simulink model "MPC_Quad_4SV_backup_before_refine"  (R2022b)
settings: Solver=FixedStepAuto  StartTime=0.0  StopTime=30  FixedStep=Ts  RelTol=1e-3
undefined symbols (not defined in the file): A, B, C, Cm, Ct, D, estim_hover_nrpm, g, initState, Ir, Ixx, Iyy, Izz, Length, mass
libraries: uavutilslib x2, sharedtransform x1, mpclib x1
settings Model: PacingRate=0.350000  Creator=Bw Jiang  LastModifiedBy=Bw Jiang
settings DebuggingCC: AlgebraicLoopMsg=none  ParameterOverflowMsg=none  ParameterUnderflowMsg=error

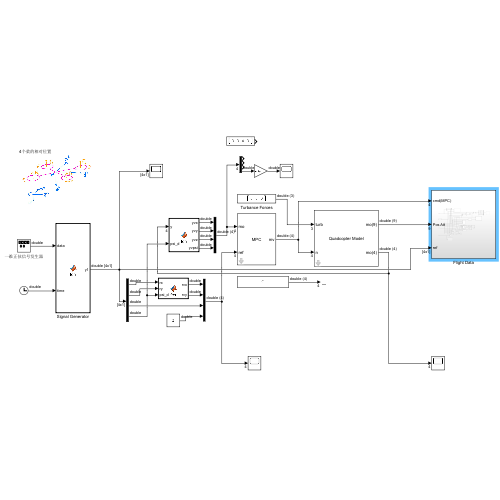
[thumbnail: Simulink's stored preview of the top-level diagram]
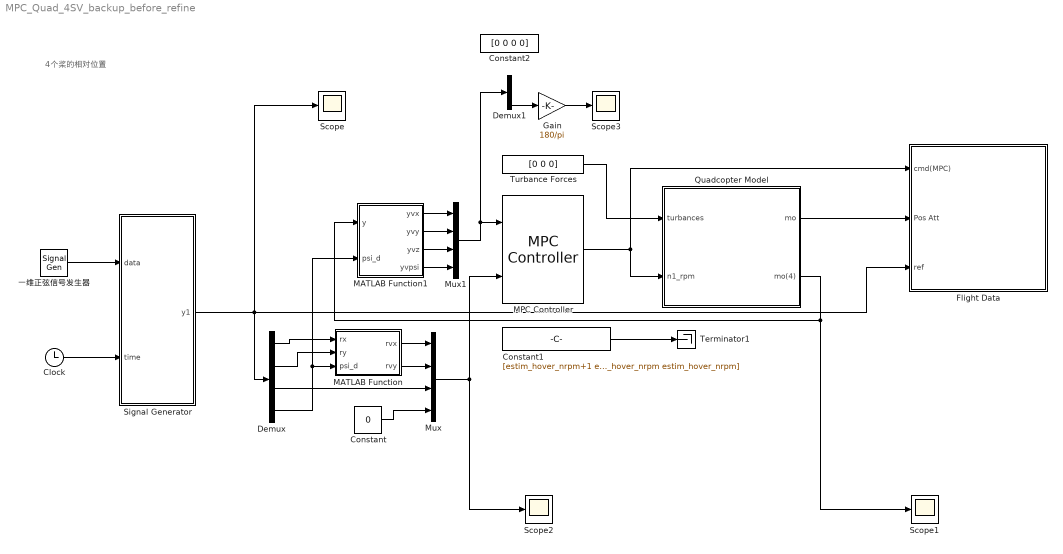
== system MPC_Quad_4SV_backup_before_refine ==
  note: 4个桨的相对位置
  Clock : Clock
  Constant : Constant  Value=0
  Constant1 : Constant  Value=[estim_hover_nrpm+1 estim_hover_nrpm estim_hover_nrpm estim_hover_nrpm]
  Constant2 : Constant  Value=[0 0 0 0]
  Demux : Demux
  Demux1 : Demux
  Flight Data : Subsystem
  Gain : Gain  Gain=180/pi
  MATLAB Function : MATLAB Function  TreatAsAtomicUnit=on
  MATLAB Function1 : MATLAB Function  TreatAsAtomicUnit=on
  MPC Controller : mpclib/MPC Controller  SCDEnableBlockLinearizationSpecification=on  mpcobj=mpc4sv  is_multiple=0  enable_value=0  return_u0=off  updateMPCinCallerWorkspace=on  md_inport=off  mv_inport=off  uref_inport=off  return_cost=off  return_mvseq=off  return_qpstatus=off  return_xseq=off  return_state=off  return_ovseq=off  state_inport=off  umin_inport=off  umax_inport=off  ymin_inport=off  ymax_inport=off  cc_inport=off  ywt_inport=off  uwt_inport=off  duwt_inport=off  rhoeps_inport=off  pm_inport=off  MaximumP=10  HorizonChoice=FixedHorizon  n_ts=0.05  n_p=30  n_mv=4  n_md=0  n_ud=0  n_mo=4  n_uo=0  BlockDataType=double  SampleTimeInherited=off  switch_inport=off
  Mux : Mux
  Mux1 : Mux
  Quadcopter Model : Subsystem  mask{g=g, mass=mass, I_xx=Ixx, I_yy=Iyy, I_zz=Izz, I_r=Ir, L=Length, C_M=Cm, C_T=Ct}
      mask prompts: g "Gravity"; I_xx "Inertia_xx"; I_yy "Inertia_yy"; I_zz "Inertia_zz"; I_r "Inertia_per_rotor"; L "Length"
      mask DialogControl ParameterGroupVar Prompt: 参数
      mask Display:
      | disp('Quadcopter Model');
      | port_label('input', 1, 'turb')
      | port_label('input', 2, 'n')
      | % port_label('input', 3, 'n3')
      | % port_label('input', 4, 'n4')
      | port_label('output', 1, 'mo(9)')
      | port_label('output', 2, 'mo(4)')
      | % port_label('output', 3, 'y')
      | % port_label('output', 4, 'vy')
      | % port_label('output', 5, 'z')
      | % port_label('output', 6, 'vz')
      | % port_label('output', 7, 'phi')
      | % port_label('output', 8, 'd_phi')
      | % port_label('output', 9, 'theta')
      | % port_label('output', 10, 'd_theta')
      | % port_label('output', 11, 'psi')
      | % port_label('output', 12, 'd_psi')
  Scope{,1..3} (4 alike) : Scope
  Signal Generator : MATLAB Function  TreatAsAtomicUnit=on
  Terminator1 : Terminator
  Turbance Forces : Constant  Value=[0 0 0]
  一维正弦信号发生器 : SignalGenerator  Frequency=0.01
  wires:
  Clock/1 -> Signal Generator/2(time)
  MPC Controller/1 -> Flight Data/1(cmd(MPC)), Quadcopter Model/2(n1_rpm)
  Constant1/1 -> Terminator1/1
  Quadcopter Model/1(mo) -> Flight Data/2(Pos Att)
  Quadcopter Model/2(mo(4)) -> MATLAB Function1/1(y), Scope1/1
  一维正弦信号发生器/1 -> Signal Generator/1(data)
  Turbance Forces/1 -> Quadcopter Model/1(turbances)
  Signal Generator/1(y1) -> Flight Data/3(ref), Demux/1, Scope/1
  Demux/3 -> Mux/3
  Constant/1 -> Mux/4
  Demux/1 -> MATLAB Function/1(rx)
  Demux/2 -> MATLAB Function/2(ry)
  Demux/4 -> MATLAB Function1/2(psi_d), MATLAB Function/3(psi_d)
  MATLAB Function/1(rvx) -> Mux/1
  MATLAB Function/2(rvy) -> Mux/2
  Mux/1 -> MPC Controller/2, Scope2/1
  MATLAB Function1/1(yvx) -> Mux1/1
  MATLAB Function1/2(yvy) -> Mux1/2
  MATLAB Function1/3(yvz) -> Mux1/3
  MATLAB Function1/4(yvpsi) -> Mux1/4
  Mux1/1 -> Demux1/1, MPC Controller/1
  Demux1/4 -> Gain/1
  Gain/1 -> Scope3/1

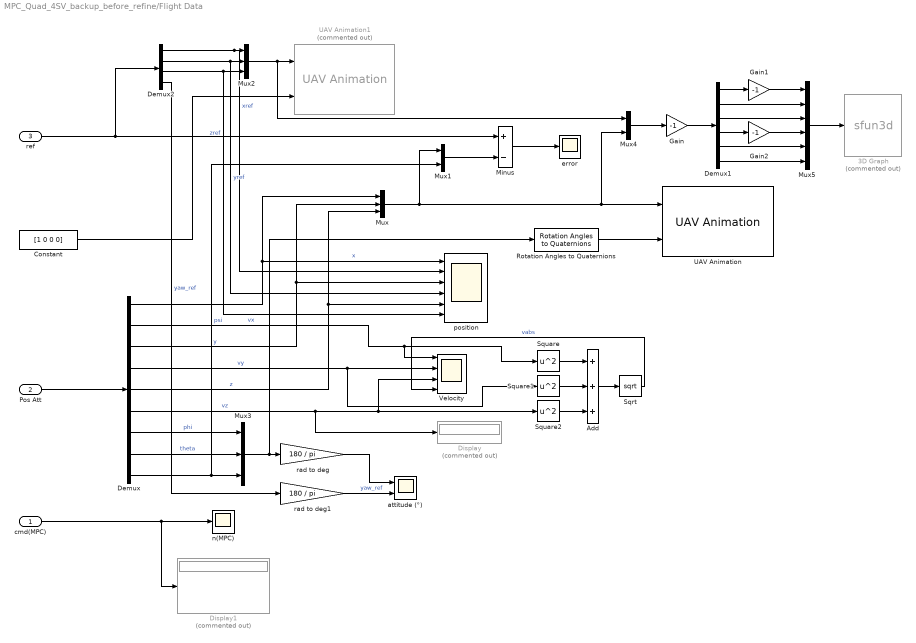
== system MPC_Quad_4SV_backup_before_refine/Flight Data ==
  cmd(MPC) : Inport
  Pos Att : Inport  Port=2
  ref : Inport  Port=3
  3D Graph : S-Function  Commented=on  LoadFcn=if exist('sfun3d','file'), sfun3d([],[],[],'LoadBlock'); end  FunctionName=sfun3d  Parameters=ax,T,np,cp,gd,ls,mk,mx,hd,tb  SFunctionDeploymentMode=off  EnableBusSupport=off  mask(3D Graph){np=2, ax=[-20 10 -10 10 -20 5], mx=50000, T=0.1, cp=[20 40 30], gd=on, hd=on, tb=on, ls=-, mk=none}
      mask prompts: np "Number of moving points (lines)"; ax "Range: [xmin xmax  ymin ymax zmin zmax]"; mx "Max number of points in each line"; T "Sampling Time"; cp "Camera position (use [0 0 1] for 2D XY view)"; gd "Grid (on|off)"; hd "HeadMarkers (on|off)"; tb "Toolbar (on|off)"; ls "LineStyle"; mk "LineMarker"
      mask help:
      | This block plots the position of several points in the XYZ space. The input contains the coordinates of all the points (x1,y1,z1,x2,y2,z2,...).
      | The number of moving points (lines), the XYZ ranges, sampling time, camera position, and grid (among other things) can be set as mask parameters.
      settings: CopyFcn=if exist('sfun3d','file'), sfun3d([],[],[],'CopyBlock'); end  DeleteFcn=if exist('sfun3d','file'), sfun3d([],[],[],'DeleteBlock'); end  NameChangeFcn=if exist('sfun3d','file'), sfun3d([],[],[],'NameChange'); end
      mask Help:
      | This block plots the position of several points in the XYZ space. The input contains the coordinates of all the points (x1,y1,z1,x2,y2,z2,...).
      | The number of moving points (lines), the XYZ ranges, sampling time, camera position, and grid (among other things) can be set as mask parameters.
      mask TypeOptions ls: - | -- | : | -. | none
      mask TypeOptions mk: none | . | + | o | * | x | square | diamond | v | ^ | > | < | pentagram | hexagram
      mask Display: plot([.05 .95 .95 .05 .05],[.45 .45 .95 .95 .45], 0.5+cos(0:0.1:2*pi)*0.3,0.7+sin(0:0.1:2*pi)*0.2)
  Add : Sum  Inputs=+++
  Constant : Constant  Value=[1 0 0 0]
  Demux : Demux  Outputs=9
  Demux1 : Demux  Outputs=6
  Demux2 : Demux
  Display : Display  Commented=on
  Display1 : Display  Commented=on
  Gain : Gain  Gain=-1
  Gain1 : Gain  Gain=-1
  Gain2 : Gain  Gain=-1
  Minus : Sum  Inputs=+-
  Mux : Mux  Inputs=3
  Mux1 : Mux  Inputs=2
  Mux2 : Mux  Inputs=3
  Mux3 : Mux  Inputs=3
  Mux4 : Mux  Inputs=2
  Mux5 : Mux  Inputs=6
  Rotation Angles to Quaternions : sharedtransform/Rotation Angles to Quaternions  rotationOrder=XYZ  aMode=aMode
  Sqrt : Sqrt
  Square : Math  Operator=square
  Square1 : Math  Operator=square
  Square2 : Math  Operator=square
  UAV Animation : uavutilslib/UAV Animation  UAVType=Multirotor  UAVSize=1  InertialZDirection=Down  SampleTime=-1
  UAV Animation1 : uavutilslib/UAV Animation  Commented=on  UAVType=Multirotor  UAVSize=1  InertialZDirection=Down  SampleTime=-1
  Velocity : Scope  NumInputPorts=4
  attitude (°) : Scope  NumInputPorts=2
  error : Scope
  n(MPC) : Scope
  position : Scope  NumInputPorts=6
  rad to deg : Gain  Gain=180 / pi
  rad to deg1 : Gain  Gain=180 / pi
  wires:
  Demux/8 -> Mux3/2  "theta"
  Demux/4 -> Square1/1, Velocity/2  "vy"
  Demux/2 -> Velocity/1, Square/1  "vx"
  Demux/7 -> Mux3/1  "phi"
  Demux/6 -> Velocity/3, Square2/1, Display/1  "vz"
  Demux/5 -> Mux/3, position/5  "z"
  Demux/1 -> Mux/1, position/1  "x"
  Demux/3 -> position/3, Mux/2  "y"
  rad to deg/1 -> attitude (°)/1
  Mux3/1 -> Rotation Angles to Quaternions/1, rad to deg/1
  cmd(MPC)/1 -> n(MPC)/1, Display1/1
  Pos Att/1 -> Demux/1
  Demux/9 -> Mux1/2, Mux3/3  "psi"
  Mux/1 -> Mux4/2, UAV Animation/1, Mux1/1
  Constant/1 -> UAV Animation1/2
  Mux1/1 -> Minus/2
  Minus/1 -> error/1
  ref/1 -> Demux2/1, Minus/1
  Demux2/1 -> position/2, Mux2/1  "xref"
  Demux2/2 -> position/4, Mux2/2  "yref"
  Demux2/3 -> position/6, Mux2/3  "zref"
  Mux2/1 -> Mux4/1, UAV Animation1/1
  Square/1 -> Add/1
  Square1/1 -> Add/2
  Square2/1 -> Add/3
  Add/1 -> Sqrt/1
  Sqrt/1 -> Velocity/4  "vabs"
  Mux4/1 -> Gain/1
  Gain/1 -> Demux1/1
  Demux1/1 -> Gain1/1
  Demux1/4 -> Gain2/1
  Gain1/1 -> Mux5/1
  Demux1/2 -> Mux5/2
  Demux1/3 -> Mux5/3
  Gain2/1 -> Mux5/4
  Demux1/5 -> Mux5/5
  Demux1/6 -> Mux5/6
  Mux5/1 -> 3D Graph/1
  Demux2/4 -> rad to deg1/1  "yaw_ref"
  rad to deg1/1 -> attitude (°)/2  "yaw_ref"
  Rotation Angles to Quaternions/1 -> UAV Animation/2

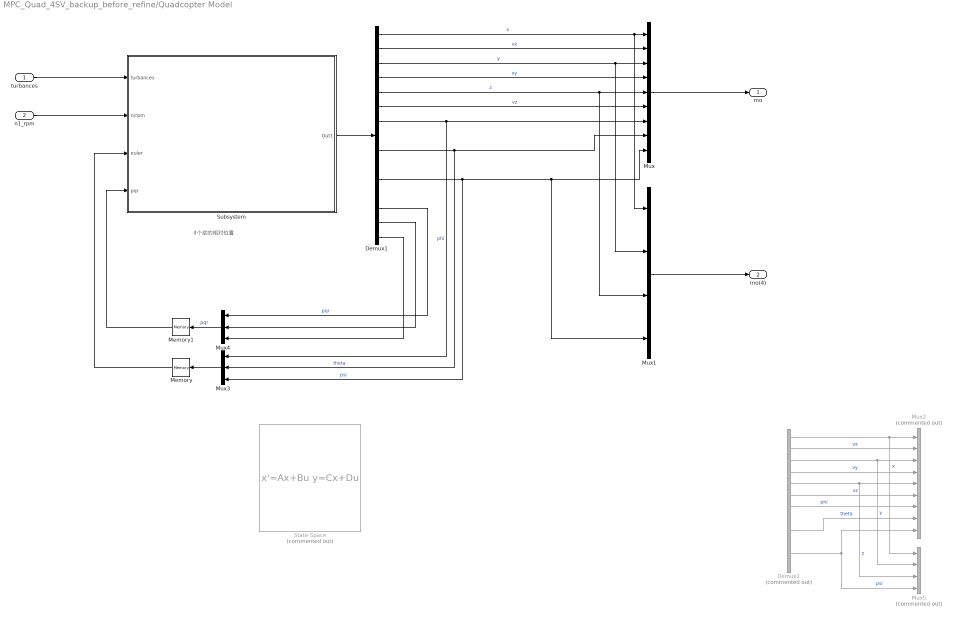
== system MPC_Quad_4SV_backup_before_refine/Quadcopter Model ==
  note: 4个桨的相对位置
  turbances : Inport
  n1_rpm : Inport  Port=2
  Demux1 : Demux  Outputs=15
  Demux2 : Demux  Commented=on  Outputs=12
  Memory : Memory  InheritSampleTime=on
  Memory1 : Memory  InheritSampleTime=on
  Mux : Mux  Inputs=9
  Mux1 : Mux
  Mux2 : Mux  Commented=on  Inputs=9
  Mux3 : Mux  Inputs=3
  Mux4 : Mux  Inputs=3
  Mux5 : Mux  Commented=on
  State-Space : StateSpace  Commented=on  A=A  B=B  C=C  D=D  InitialCondition=0
  Subsystem : Subsystem
  mo : Outport
  mo(4) : Outport  Port=2
  wires:
  n1_rpm/1 -> Subsystem/2(n/rpm)
  Memory1/1 -> Subsystem/4(pqr)
  Demux1/15 -> Mux4/3
  Demux1/13 -> Mux4/1  "pqr"
  Mux4/1 -> Memory1/1  "pqr"
  Demux1/9 -> Mux/8, Mux3/2  "theta"
  Demux1/1 -> Mux1/1, Mux/1  "x"
  Demux1/2 -> Mux/2  "vx"
  Demux1/11 -> Mux1/4, Mux/9, Mux3/3  "psi"
  Demux1/4 -> Mux/4  "vy"
  Demux1/3 -> Mux1/2, Mux/3  "y"
  Demux1/5 -> Mux1/3, Mux/5  "z"
  Subsystem/1(Out1) -> Demux1/1
  Memory/1 -> Subsystem/3(euler)
  Demux1/6 -> Mux/6  "vz"
  Demux1/7 -> Mux/7, Mux3/1  "phi"
  Mux3/1 -> Memory/1
  Demux1/14 -> Mux4/2
  turbances/1 -> Subsystem/1(turbances)
  Demux2/1 -> Mux2/1, Mux5/1  "x"
  Demux2/2 -> Mux2/2  "vx"
  Demux2/3 -> Mux5/2, Mux2/3  "y"
  Demux2/4 -> Mux2/4  "vy"
  Demux2/5 -> Mux5/3, Mux2/5  "z"
  Demux2/6 -> Mux2/6  "vz"
  Demux2/7 -> Mux2/7  "phi"
  Demux2/9 -> Mux2/8  "theta"
  Demux2/11 -> Mux5/4, Mux2/9  "psi"
  Mux/1 -> mo/1
  Mux1/1 -> mo(4)/1

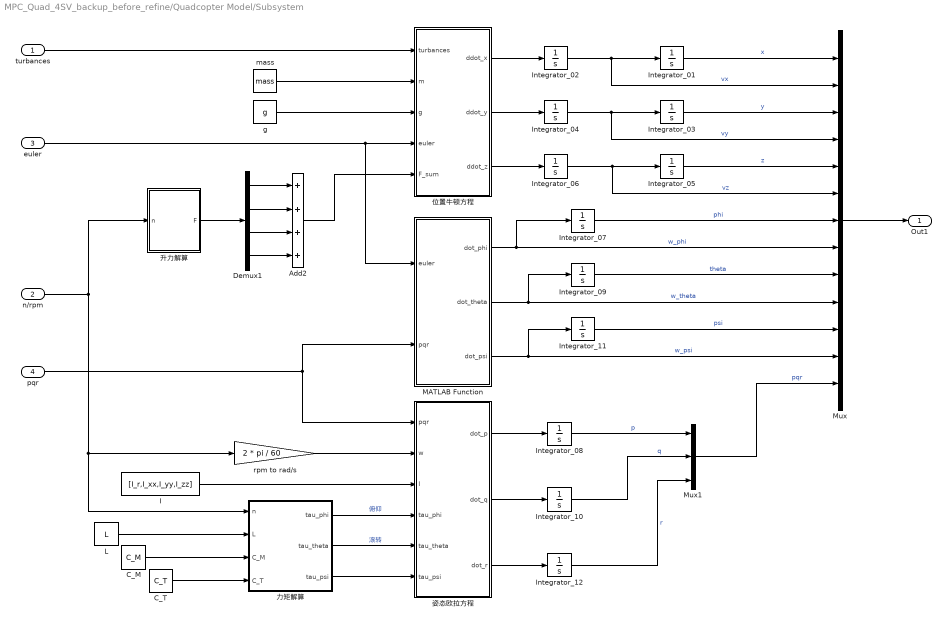
== system MPC_Quad_4SV_backup_before_refine/Quadcopter Model/Subsystem ==
  turbances : Inport
  n/rpm : Inport  Port=2  PortDimensions=4
  euler : Inport  Port=3  PortDimensions=3
  pqr : Inport  Port=4  PortDimensions=3
  Add2 : Sum  Inputs=++++
  C_M : Constant  Value=C_M
  C_T : Constant  Value=C_T
  Demux1 : Demux
  I : Constant  Value=[I_r,I_xx,I_yy,I_zz]
  Integrator_01 : Integrator  InitialCondition=initState.x
  Integrator_02 : Integrator  InitialCondition=initState.vx
  Integrator_03 : Integrator  InitialCondition=initState.y
  Integrator_04 : Integrator  InitialCondition=initState.vy
  Integrator_05 : Integrator  InitialCondition=initState.z
  Integrator_06 : Integrator  InitialCondition=initState.vz
  Integrator_07 : Integrator  InitialCondition=initState.phi
  Integrator_08 : Integrator  InitialCondition=initState.p
  Integrator_09 : Integrator  InitialCondition=initState.theta
  Integrator_10 : Integrator  InitialCondition=initState.q
  Integrator_11 : Integrator  InitialCondition=initState.psi
  Integrator_12 : Integrator  InitialCondition=initState.r
  L : Constant  Value=L
  MATLAB Function : MATLAB Function  TreatAsAtomicUnit=on
  Mux : Mux  Inputs=13
  Mux1 : Mux  Inputs=3
  g : Constant  Value=g
  mass : Constant  Value=mass
  rpm to rad/s : Gain  Gain=2 * pi / 60
  位置牛顿方程 : MATLAB Function  TreatAsAtomicUnit=on
  力矩解算 : MATLAB Function  TreatAsAtomicUnit=on
  升力解算 : MATLAB Function  TreatAsAtomicUnit=on
  姿态欧拉方程 : MATLAB Function  TreatAsAtomicUnit=on
  Out1 : Outport
  wires:
  姿态欧拉方程/1(dot_p) -> Integrator_08/1
  Demux1/4 -> Add2/4
  pqr/1 -> MATLAB Function/2(pqr), 姿态欧拉方程/1(pqr)
  位置牛顿方程/2(ddot_y) -> Integrator_04/1
  姿态欧拉方程/2(dot_q) -> Integrator_10/1
  I/1 -> 姿态欧拉方程/3(I)
  位置牛顿方程/3(ddot_z) -> Integrator_06/1
  Mux/1 -> Out1/1
  g/1 -> 位置牛顿方程/3(g)
  位置牛顿方程/1(ddot_x) -> Integrator_02/1
  Integrator_10/1 -> Mux1/2  "q"
  Demux1/1 -> Add2/1
  力矩解算/1(tau_phi) -> 姿态欧拉方程/4(tau_phi)  "俯仰"
  Integrator_08/1 -> Mux1/1  "p"
  euler/1 -> MATLAB Function/1(euler), 位置牛顿方程/4(euler)
  Integrator_03/1 -> Mux/3  "y"
  Integrator_09/1 -> Mux/9  "theta"
  力矩解算/3(tau_psi) -> 姿态欧拉方程/6(tau_psi)
  Demux1/2 -> Add2/2
  Add2/1 -> 位置牛顿方程/5(F_sum)
  Integrator_12/1 -> Mux1/3  "r"
  mass/1 -> 位置牛顿方程/2(m)
  力矩解算/2(tau_theta) -> 姿态欧拉方程/5(tau_theta)  "滚转"
  Demux1/3 -> Add2/3
  Integrator_05/1 -> Mux/5  "z"
  Integrator_01/1 -> Mux/1  "x"
  Integrator_02/1 -> Integrator_01/1, Mux/2  "vx"
  Integrator_07/1 -> Mux/7  "phi"
  Integrator_04/1 -> Mux/4, Integrator_03/1  "vy"
  Integrator_06/1 -> Mux/6, Integrator_05/1  "vz"
  Integrator_11/1 -> Mux/11  "psi"
  姿态欧拉方程/3(dot_r) -> Integrator_12/1
  MATLAB Function/3(dot_psi) -> Integrator_11/1, Mux/12  "w_psi"
  MATLAB Function/2(dot_theta) -> Integrator_09/1, Mux/10  "w_theta"
  MATLAB Function/1(dot_phi) -> Integrator_07/1, Mux/8  "w_phi"
  Mux1/1 -> Mux/13  "pqr"
  升力解算/1(F) -> Demux1/1
  L/1 -> 力矩解算/2(L)
  n/rpm/1 -> 升力解算/1(n), rpm to rad/s/1, 力矩解算/1(n)
  rpm to rad/s/1 -> 姿态欧拉方程/2(w)
  C_M/1 -> 力矩解算/3(C_M)
  C_T/1 -> 力矩解算/4(C_T)
  turbances/1 -> 位置牛顿方程/1(turbances)

== matlab function MPC_Quad_4SV_backup_before_refine/Quadcopter Model/Subsystem/MATLAB Function ==
  data: euler input; pqr input; dot_phi output; dot_theta output; dot_psi output
function [dot_phi, dot_theta, dot_psi] = fcn(euler, pqr)

% 角加速度的坐标转换，从机体系b到惯性系e

p = pqr(1);
q = pqr(2);
r = pqr(3);

phi =euler(1);
theta = euler(2);
psi = euler(3);

mat = [
    1, tan(theta) * sin(phi), tan(theta) * cos(phi);
    0, cos(phi), -sin(phi);
    0, sin(phi) / cos(theta), cos(phi) / cos(theta)
    ];
body = [p; q; r];
earth = mat * body;

dot_phi = earth(1);
dot_theta = earth(2);
dot_psi = earth(3);

== matlab function MPC_Quad_4SV_backup_before_refine/Quadcopter Model/Subsystem/位置牛顿方程 ==
  data: turbances input; m input; g input; euler input; ddot_x output; F_sum input; ddot_y output; ddot_z output
function [ddot_x, ddot_y, ddot_z] = fcn(turbances, m, g, euler, F_sum)

% F_sum恒正

phi =euler(1);
theta = euler(2);
psi = euler(3);

ddot_x = -((cos(phi) * sin(theta) * cos(psi) + sin(phi) * sin(psi)) * F_sum + turbances(1)) / m;
ddot_y = -((cos(phi) * sin(theta) * sin(psi) - sin(phi) * cos(psi)) * F_sum + turbances(2)) / m;
ddot_z = -(cos(phi) * cos(theta) * F_sum + turbances(3)) / m + g;

end

== matlab function MPC_Quad_4SV_backup_before_refine/Quadcopter Model/Subsystem/姿态欧拉方程 ==
  data: pqr input; dot_p output; w input; I input; dot_q output; dot_r output; tau_phi input; tau_theta input; tau_psi input
function [dot_p, dot_q, dot_r] = fcn(pqr, w, I, tau_phi, tau_theta, tau_psi)

w1 = w(1);
w2 = w(2);
w3 = w(3);
w4 = w(4);

p = pqr(1);
q = pqr(2);
r = pqr(3);

I_r = I(1);
I_xx = I(2);
I_yy = I(3);
I_zz = I(4);

w_tau = w1 - w2 + w3 - w4;

dot_p = (I_yy - I_zz) / I_xx * q * r - I_r * q / I_xx * w_tau + tau_phi / I_xx;
dot_q = (I_zz - I_xx) / I_yy * p * r + I_r * p / I_yy * w_tau + tau_theta / I_yy;
dot_r = (I_xx - I_yy) / I_zz * q * p + tau_psi / I_zz;

end

== matlab function MPC_Quad_4SV_backup_before_refine/Quadcopter Model/Subsystem/升力解算 ==
  data: n input; F output
function F = fcn(n)
%% Input Vars
% n - rpm

%% Output Vars
% F - N

%% Mid Vars
% omega - rad/s

%% Code

% F = n .* n * 2.414e-7 * 2;

omega = n / 60 * 2 * pi;
F = omega .* omega * 1.11e-5;

end

== matlab function MPC_Quad_4SV_backup_before_refine/Signal Generator ==
  data: data input; time input; y1 output
function y1  = fcn(data, time)

starttime = 2;

%% 悬停

% y1 = [0
%         0
%         0
%         0];

%% 螺旋线轨迹

% radspeed = 45; % 相当于相对圆心角的角速度 °/s
% vz = 0;
% r = 2 + time * 0.0;
% if time < starttime
%     y1 = [0
%           0
%           0
%           0];
% else
%     if r > 15
%         r = 15;
%     end
%     y1 = [r - r * cos(radspeed * (time - starttime) * pi / 180)
%           r * sin(radspeed * (time - starttime) * pi / 180)
%           -vz * time
%           0];
% end

%% 类8字轨迹

% radspeed = 10; % 相当于相对圆心角的角速度 °/s
% vz = 0.2;
% r1 = 4;
% r2 = 8;
% if time < starttime
%     y1 = [0; 0; 0; 0];
% else
%     if time < starttime + 180 / radspeed
%         y1 = [r1 - r1 * cos(radspeed * (time - starttime) * pi / 180)
%               r1 * sin(radspeed * (time - starttime) * pi / 180)
%               vz * (time - starttime)
%               0];
%     else
%         if time < starttime + 360 / radspeed
%             y1 = [-r2 * cos(radspeed * (time - starttime) * pi / 180)
%                   r2 * sin(radspeed * (time - starttime) * pi / 180)
%                   vz * (time - starttime)
%                   0];
%         else
%             if time < starttime + 540 / radspeed
%                 y1 = [-(r1 + r2) + r1 * cos(- radspeed * (time - starttime - 360 / radspeed) * pi / 180)
%                       r1 * sin(radspeed * (time - starttime) * pi / 180)
%                       vz * 360 / radspeed - vz * (time - starttime - 360 / radspeed)
%                       0];
%             else
%                 if time < starttime + 720 / radspeed
%                     y1 = [-r2 + r2 * cos(2 * pi - radspeed * (time - starttime - 360 / radspeed) * pi / 180)
%                           r2 * sin(radspeed * (time - starttime - 360 / radspeed) * pi / 180)
%                           vz * 360 / radspeed - vz * (time - starttime - 360 / radspeed)
%                           0];
%                 else
%                     y1 = [0; 0; 0; 0];
%                 end
%             end
%         end
%     end
% end

%% 阶跃轨迹

% x = 0;
% y = 0;
% z = 0;
% yaw = 0;
% 
% if time < 10
%     x = 0;
%     y = 0;
%     z = 0;
%     yaw = 0;
% elseif time > 10
%     x = 1;
%     y = 1.2;
%     z = -0.8;
%     yaw = 0;
% end
% 
% y1 = [x
%     y
%     z
%     yaw];

%% 偏航控制测试

yawspeed = 10; % °/s
yawspeed = yawspeed * pi / 180; % rad/s

t1 = starttime + 3;
t2 = t1 + 20;
t3 = t2 + 4;
t4 = t3 + 7;
t5 = t4 + 7;
if time < starttime
    y1 = [0
          0
          0
          0];
else
    if time < t1
    y1 = [0
          0
          0
          yawspeed * (time - starttime)];
    else
        if time < t2
            y1 = [0
                  0
                  0
                  yawspeed * (t1 - starttime)];
        else
            if time < t3
                y1 = [0
                      0
                      0
                      yawspeed * (time - t2 + t1 - starttime)];
            else
                if time < t4
                    y1 = [0
                          0
                          0
                          yawspeed * (t3 - t2 + t1 - starttime)];

                else
                    if time < t5
                        y1 = [0
                              0
                              0
                              yawspeed * (t3 - t2 + t1 - starttime) / (t4 - t5) * (time - t5)];
                    else
                        y1 = [0
                              0
                              0
                              0];
                    end
                end
            end
        end
    end
end

end

== matlab function MPC_Quad_4SV_backup_before_refine/Quadcopter Model/Subsystem/力矩解算 ==
  data: n input; L input; tau_phi output; tau_theta output; tau_psi output; C_M input; C_T input
function [tau_phi, tau_theta, tau_psi]= fcn(n, L, C_M, C_T)
%% Input Vars
% n - rpm
% L - m
% C_M - N*m*s^2/rad^2
% C_T - N*s^2/rad^2

%% Output Vars
% tau - N*m

%% Mid Vars
% w - rad/s

%% Code

% C_T = 1.1e-5;
% C_M = 1.0144e-7;

% F1 = F(1);
% F2 = F(2);
% F3 = F(3);
% F4 = F(4);

w1 = n(1) / 60 * 2 * pi;
w2 = n(2) / 60 * 2 * pi;
w3 = n(3) / 60 * 2 * pi;
w4 = n(4) / 60 * 2 * pi;

% I_r = I(1);

% w_tau = w1 + w3 - w2 - w4;

% 横滚
tau_phi = sqrt(2) / 2 * C_T * L * (w1^2 - w2^2 - w3^2 + w4^2); % tau_phi = (F1+F2-F3-F4) * L;
% 俯仰
tau_theta = sqrt(2) / 2 * C_T * L * (w1^2 + w2^2 - w3^2 - w4^2); % tau_theta = (F1-F2-F3+F4) * L;
% 偏航
tau_psi = C_M * (w1^2 - w2^2 + w3^2 - w4^2); % tau_psi = w_tau * I_r;

end

== matlab function MPC_Quad_4SV_backup_before_refine/MATLAB Function ==
  data: rx input; rvx output; ry input; psi_d input; rvy output
function [rvx, rvy] = fcn(rx, ry, psi_d)

rvx = rx * cos(psi_d) - ry * sin(psi_d);
rvy = rx * sin(psi_d) + ry * cos(psi_d);

end

== matlab function MPC_Quad_4SV_backup_before_refine/MATLAB Function1 ==
  data: y input; yvx output; psi_d input; yvy output; yvz output; yvpsi output
function [yvx, yvy, yvz, yvpsi] = fcn(y, psi_d)

yx = y(1);
yy = y(2);
yz = y(3);
ypsi = y(4);

yvx = yx * cos(psi_d) - yy * sin(psi_d);
yvy = yx * sin(psi_d) + yy * cos(psi_d);
yvz = yz;
yvpsi = ypsi - psi_d;

end
